simulink subsystem "block_environment"  (R2019b)
settings: Solver=VariableStepAuto  StartTime=0.0  StopTime=10.0  RelTol=1e-3
undefined symbols (not defined in the file): r, RP
libraries: blocklib x10, aerolibconvert2 x1
settings Model: Creator=imanol  LastModifiedBy=imanol

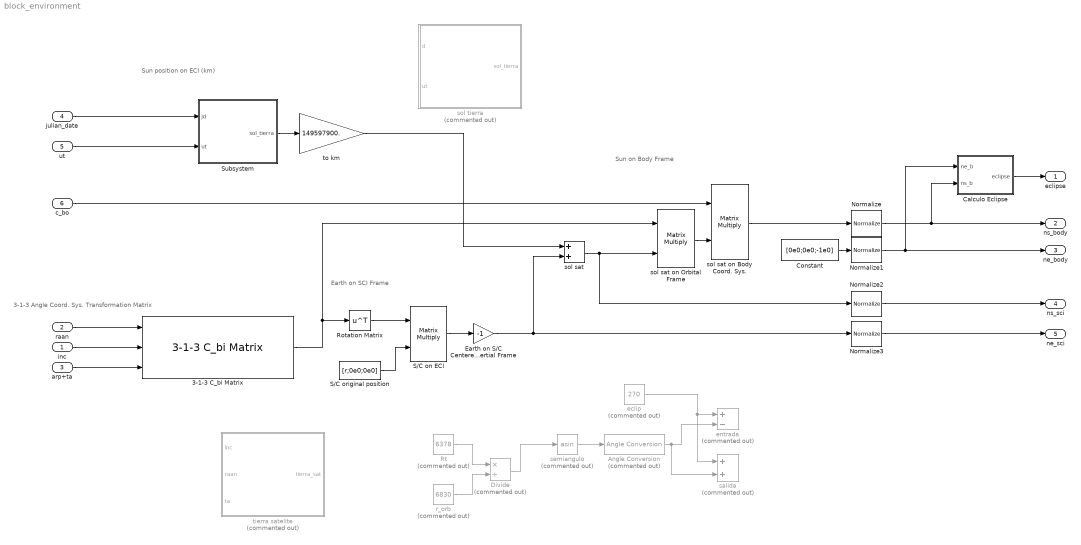
== system block_environment ==
  note: Earth on SCI Frame
  note: Sun on Body Frame
  note: Sun position on ECI (km)
  note: 3-1-3 Angle Coord. Sys. Transformation Matrix
  inc : Inport
  raan : Inport  Port=2
  arp+ta : Inport  Port=3
  julian_date : Inport  Port=4
  ut : Inport  Port=5
  c_bo : Inport  Port=6
  3-1-3 C_bi Matrix : blocklib/3-1-3 C_bi Matrix  SystemSampleTime=-1  Latency=0  AutoFrameSizeCalculation=off
      settings: SourceProductName=Custom Library
  Angle Conversion : aerolibconvert2/Angle Conversion  Commented=on  IU=rad  OU=deg
  Calculo Eclipse : Subsystem
  Constant : Constant  Value=[0e0;0e0;-1e0]
  Divide : Product  Commented=on  Inputs=*/
  Earth on S/C Centered Inertial Frame : Gain  Gain=-1
  Normalize{,1..3} (4 alike) : blocklib/Normalize  SystemSampleTime=-1  Latency=0  AutoFrameSizeCalculation=off
      settings: SourceProductName=Custom Library
  Rotation Matrix : Math  Operator=transpose  SignedPower=off  SaturateOnIntegerOverflow=on
  Rt : Constant  Commented=on  Value=6378
  S/C on ECI : Product  Multiplication=Matrix(*)
  S/C original position : Constant  Value=[r;0e0;0e0]
  Subsystem : Subsystem
  eclip : Constant  Commented=on  Value=270
  entrada : Sum  Commented=on  Inputs=+-
  r_orb : Constant  Commented=on  Value=6830
  salida : Sum  Commented=on
  semiangulo : Trigonometry  Commented=on  Operator=asin
  sol sat : Sum
  sol sat on Body Coord. Sys. : Product  Multiplication=Matrix(*)
  sol sat on Orbital Frame : Product  Multiplication=Matrix(*)
  sol tierra : MATLAB Function  Commented=on  TreatAsAtomicUnit=on
  tierra satelite : MATLAB Function  Commented=on  TreatAsAtomicUnit=on
  to km : Gain  Gain=149597900.
  eclipse : Outport  VectorParamsAs1DForOutWhenUnconnected=off
  ns_body : Outport  Port=2  VectorParamsAs1DForOutWhenUnconnected=off
  ne_body : Outport  Port=3  VectorParamsAs1DForOutWhenUnconnected=off
  ns_sci : Outport  Port=4  VectorParamsAs1DForOutWhenUnconnected=off
  ne_sci : Outport  Port=5  VectorParamsAs1DForOutWhenUnconnected=off
  wires:
  raan/1 -> 3-1-3 C_bi Matrix/1
  arp+ta/1 -> 3-1-3 C_bi Matrix/3
  Divide/1 -> semiangulo/1
  Rt/1 -> Divide/1
  r_orb/1 -> Divide/2
  inc/1 -> 3-1-3 C_bi Matrix/2
  eclip/1 -> salida/1, entrada/1
  Angle Conversion/1 -> salida/2, entrada/2
  ut/1 -> Subsystem/2(ut)
  julian_date/1 -> Subsystem/1(jd)
  semiangulo/1 -> Angle Conversion/1
  Constant/1 -> Normalize1/1
  3-1-3 C_bi Matrix/1 -> sol sat on Orbital Frame/1, Rotation Matrix/1
  sol sat on Orbital Frame/1 -> sol sat on Body Coord. Sys./2
  c_bo/1 -> sol sat on Body Coord. Sys./1
  sol sat on Body Coord. Sys./1 -> Normalize/1
  Calculo Eclipse/1(eclipse) -> eclipse/1
  S/C original position/1 -> S/C on ECI/2
  Rotation Matrix/1 -> S/C on ECI/1
  S/C on ECI/1 -> Earth on S/C Centered Inertial Frame/1
  Earth on S/C Centered Inertial Frame/1 -> Normalize3/1, sol sat/2
  sol sat/1 -> sol sat on Orbital Frame/2, Normalize2/1
  Normalize/1 -> ns_body/1, Calculo Eclipse/2(ns_b)
  to km/1 -> sol sat/1
  Subsystem/1(sol_tierra) -> to km/1
  Normalize1/1 -> Calculo Eclipse/1(ne_b), ne_body/1
  Normalize2/1 -> ns_sci/1
  Normalize3/1 -> ne_sci/1

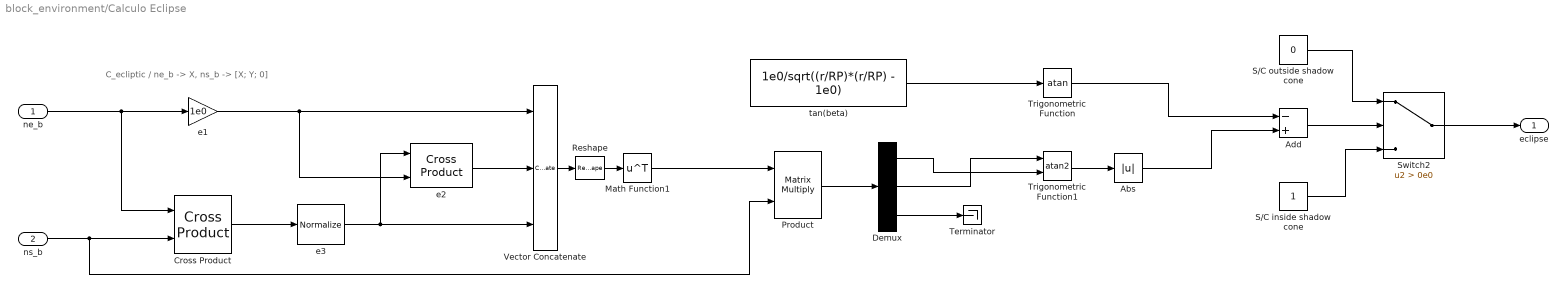
== system block_environment/Calculo Eclipse ==
  note: C_ecliptic / ne_b -> X, ns_b -> [X; Y; 0]
  ne_b : Inport
  ns_b : Inport  Port=2
  Abs : Abs
  Add : Sum  Inputs=-+
  Cross Product : blocklib/Cross Product  SystemSampleTime=-1  Latency=0  AutoFrameSizeCalculation=off
      settings: SourceProductName=Custom Library
  Demux : Demux  Outputs=3
  Math Function1 : Math  Operator=transpose  SignedPower=off  SaturateOnIntegerOverflow=on
  Product : Product  Multiplication=Matrix(*)
  Reshape : Reshape  OutputDimensionality=Customize  OutputDimensions=[3,3]
  S/C inside shadow cone : Constant
  S/C outside shadow cone : Constant  Value=0
  Switch2 : Switch  Criteria=u2 > Threshold  Threshold=0e0
  Terminator : Terminator
  Trigonometric Function : Trigonometry  Operator=atan
  Trigonometric Function1 : Trigonometry  Operator=atan2
  Vector Concatenate : Concatenate  NumInputs=3
  e1 : Gain  Gain=1e0
  e2 : blocklib/Cross Product  SystemSampleTime=-1  Latency=0  AutoFrameSizeCalculation=off
      settings: SourceProductName=Custom Library
  e3 : blocklib/Normalize  SystemSampleTime=-1  Latency=0  AutoFrameSizeCalculation=off
      settings: SourceProductName=Custom Library
  tan(beta) : Constant  Value=1e0/sqrt((r/RP)*(r/RP) - 1e0)
  eclipse : Outport
  wires:
  Switch2/1 -> eclipse/1
  Trigonometric Function/1 -> Add/1
  Abs/1 -> Add/2
  Add/1 -> Switch2/2
  Trigonometric Function1/1 -> Abs/1
  S/C inside shadow cone/1 -> Switch2/3
  S/C outside shadow cone/1 -> Switch2/1
  Demux/1 -> Trigonometric Function1/2
  Demux/2 -> Trigonometric Function1/1
  Demux/3 -> Terminator/1
  Product/1 -> Demux/1
  Math Function1/1 -> Product/1
  Reshape/1 -> Math Function1/1
  Vector Concatenate/1 -> Reshape/1
  e2/1 -> Vector Concatenate/2
  e1/1 -> e2/2, Vector Concatenate/1
  e3/1 -> Vector Concatenate/3, e2/1
  Cross Product/1 -> e3/1
  ns_b/1 -> Product/2, Cross Product/2
  tan(beta)/1 -> Trigonometric Function/1
  ne_b/1 -> e1/1, Cross Product/1

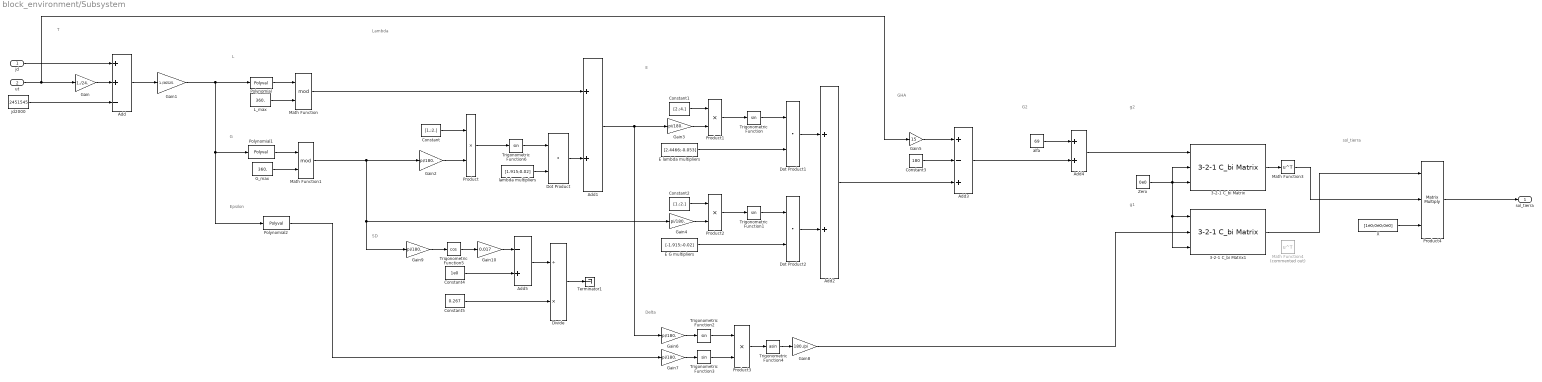
== system block_environment/Subsystem ==
  note: T
  note: L
  note: G
  note: Lambda
  note: Epsilon
  note: E
  note: GHA
  note: Delta
  note: G2
  note: SD
  note: g2
  note: g1
  note: sol_tierra
  jd : Inport
  ut : Inport  Port=2
  3-2-1 C_bi Matrix : blocklib/3-2-1 C_bi Matrix  Tag=|  SystemSampleTime=-1  Latency=0  AutoFrameSizeCalculation=off
      | text(.05,.5,'{\itEquation:}  \Sigma \alpha^2 + 
      | \beta^2 \rightarrow \infty, \Pi, \phi_3 = {\bfcool}', 
      | 'hor','left','texmode','on')
      settings: SourceProductName=Custom Library
  3-2-1 C_bi Matrix1 : blocklib/3-2-1 C_bi Matrix  Tag=|  SystemSampleTime=-1  Latency=0  AutoFrameSizeCalculation=off
      | text(.05,.5,'{\itEquation:}  \Sigma \alpha^2 + 
      | \beta^2 \rightarrow \infty, \Pi, \phi_3 = {\bfcool}', 
      | 'hor','left','texmode','on')
      settings: SourceProductName=Custom Library
  Add : Sum  Inputs=++-
  Add1 : Sum
  Add2 : Sum
  Add3 : Sum  Inputs=+-+
  Add4 : Sum
  Add5 : Sum  Inputs=-+
  Constant : Constant  Value=[1.;2.]
  Constant1 : Constant  Value=[2.;4.]
  Constant2 : Constant  Value=[1.;2.]
  Constant3 : Constant  Value=180
  Constant4 : Constant  Value=1e0
  Constant5 : Constant  Value=0.267
  Divide : Product  Inputs=/*
  Dot Product : DotProduct  InputSameDT=on  OutDataTypeStr=Inherit: Inherit via internal rule
  Dot Product1 : DotProduct  InputSameDT=on  OutDataTypeStr=Inherit: Inherit via internal rule
  Dot Product2 : DotProduct  InputSameDT=on  OutDataTypeStr=Inherit: Inherit via internal rule
  E G multipliers : Constant  Value=[-1.915;-0.02]
  E lambda multipliers : Constant  Value=[2.4466;-0.053]
  G_max : Constant  Value=360.
  Gain : Gain  Gain=1./24.
  Gain1 : Gain  Gain=1./36525.
  Gain10 : Gain  Gain=0.017
  Gain{2..4,6..7,9} (6 alike) : Gain  Gain=pi/180.
  Gain5 : Gain  Gain=15
  Gain8 : Gain  Gain=180./pi
  L_max : Constant  Value=360.
  Math Function : Math  Operator=mod  SignedPower=off  SaturateOnIntegerOverflow=on
  Math Function1 : Math  Operator=mod  SignedPower=off  SaturateOnIntegerOverflow=on
  Math Function3 : Math  Operator=transpose  SignedPower=off  SaturateOnIntegerOverflow=on
  Math Function4 : Math  Commented=on  Operator=transpose  SignedPower=off  SaturateOnIntegerOverflow=on
  Polynomial : Polyval  Coefs=[36000.77;280.46]
  Polynomial1 : Polyval  Coefs=[35999.05;357.528]
  Polynomial2 : Polyval  Coefs=[-0.013;23.4393]
  Product{,1..3} (4 alike) : Product
  Product4 : Product  Inputs=3  Multiplication=Matrix(*)
  Terminator1 : Terminator
  Trigonometric Function{,1..3,6} (5 alike) : Trigonometry
  Trigonometric Function4 : Trigonometry  Operator=asin
  Trigonometric Function5 : Trigonometry  Operator=cos
  X : Constant  Value=[1e0;0e0;0e0]
  Zero : Constant  Value=0e0
  alfa : Constant  Value=69
  jd2000 : Constant  Value=2451545
  lambda multipliers : Constant  Value=[1.915;0.02]
  sol_tierra : Outport
  wires:
  Math Function/1 -> Add1/1
  Gain2/1 -> Product/2
  X/1 -> Product4/3
  Product4/1 -> sol_tierra/1
  3-2-1 C_bi Matrix1/1 -> Product4/1
  Math Function3/1 -> Product4/2
  3-2-1 C_bi Matrix/1 -> Math Function3/1
  Zero/1 -> 3-2-1 C_bi Matrix/3, 3-2-1 C_bi Matrix/2, 3-2-1 C_bi Matrix1/1, 3-2-1 C_bi Matrix1/3
  Gain8/1 -> 3-2-1 C_bi Matrix1/2
  Add4/1 -> 3-2-1 C_bi Matrix/1
  Divide/1 -> Terminator1/1
  Constant4/1 -> Add5/2
  Constant5/1 -> Divide/2
  Add5/1 -> Divide/1
  Gain10/1 -> Add5/1
  Trigonometric Function5/1 -> Gain10/1
  Gain9/1 -> Trigonometric Function5/1
  alfa/1 -> Add4/1
  Add3/1 -> Add4/2
  Trigonometric Function4/1 -> Gain8/1
  Product3/1 -> Trigonometric Function4/1
  Trigonometric Function3/1 -> Product3/2
  Trigonometric Function2/1 -> Product3/1
  Gain7/1 -> Trigonometric Function3/1
  Gain6/1 -> Trigonometric Function2/1
  Polynomial2/1 -> Gain7/1
  Gain5/1 -> Add3/1
  Add2/1 -> Add3/3
  Constant3/1 -> Add3/2
  Gain3/1 -> Product1/2
  Gain4/1 -> Product2/2
  Dot Product1/1 -> Add2/1
  Dot Product2/1 -> Add2/2
  Trigonometric Function1/1 -> Dot Product2/1
  Product2/1 -> Trigonometric Function1/1
  E G multipliers/1 -> Dot Product2/2
  Constant2/1 -> Product2/1
  Math Function1/1 -> Gain2/1, Gain4/1, Gain9/1
  E lambda multipliers/1 -> Dot Product1/2
  Trigonometric Function/1 -> Dot Product1/1
  Product1/1 -> Trigonometric Function/1
  Add1/1 -> Gain3/1, Gain6/1
  Constant1/1 -> Product1/1
  Dot Product/1 -> Add1/2
  lambda multipliers/1 -> Dot Product/2
  Trigonometric Function6/1 -> Dot Product/1
  Product/1 -> Trigonometric Function6/1
  Constant/1 -> Product/1
  Polynomial1/1 -> Math Function1/1
  G_max/1 -> Math Function1/2
  Gain1/1 -> Polynomial/1, Polynomial2/1, Polynomial1/1
  L_max/1 -> Math Function/2
  Polynomial/1 -> Math Function/1
  Add/1 -> Gain1/1
  jd2000/1 -> Add/3
  jd/1 -> Add/1
  Gain/1 -> Add/2
  ut/1 -> Gain/1, Gain5/1

== matlab function block_environment/sol tierra ==
  data: d input; sol_tierra output; ut input
function sol_tierra = fcn(d,ut)

% d=juliandate([2018,month,1,ut,0,0]);
% d=2458271;
T=(d+ut/24-2451545)/36525;

L=mod(280.46+36000.77*T,360);
G=mod(357.528+35999.05*T,360);
lambda=L+1.915*sind(G)+0.02*sind(2*G);
epsilon=23.4393-0.013*T;
E=-1.915*sind(G)-0.02*sind(2*G)+2.4466*sind(2*lambda)-0.053*sind(4*lambda);
GHA=15*ut-180+E;
delta=asind(sind(epsilon)*sind(lambda));
alfa=69; %angulo meridiano punto aries
g2=alfa+GHA;
SD=0.267/(1-0.017*cosd(G));

g1=[cosd(delta) 0 -sind(delta); 0 1 0;sind(delta) 0 cosd(delta)];
g2=[cosd(g2) -sind(g2) 0;sind(g2) cosd(g2) 0; 0 0 1];
v=g1*g2*[1; 0 ;0];

sol_tierra=v;

== matlab function block_environment/tierra satelite ==
  data: tierra_sat output; inc input; raan input; ta input
function tierra_sat = fcn(inc, raan, ta)

R=([cosd(raan) -sind(raan) 0; sind(raan) cosd(raan) 0; 0 0 1]*[1 0 0; 0 cosd(inc) -sind(inc);0 sind(inc) cosd(inc)]);
C_opf=R';
C_opr=[ cosd(ta) sind(ta) 0; -sind(ta) cosd(ta) 0; 0 0 1];
C_lv=[0 1 0;0 0 -1;-1 0 0];
r_lv=[0;0;1];
% r_lv=[0;0;r];
TS=C_opf*C_opr*C_lv*r_lv;


% TS=TS/norm(TS);

tierra_sat=TS;
